simulink model "simulacion_controlador_lqr_entrada_velocidad"  (R2015a)
settings: Solver=ode45  StartTime=0.0  StopTime=144  RelTol=1e-3
values from neighbouring files (symbols this model uses):
  g = 9.81    [bola_viga_funciones.m]    (also in bola_viga_vel_funciones.m)
  Ib = 0.4*m*R^2    (= 4.624e-05)    [bola_viga_funciones.m]    (also in bola_viga_vel_funciones.m)
  L1 = place(AD',(CD*AD)',Pzo)'    [bola_viga_funciones.m]    (also in bola_viga_vel_funciones.m)
  m = 0.1    [bola_viga_funciones.m]    (also in bola_viga_vel_funciones.m)
  R = 0.034    [bola_viga_funciones.m]    (also in bola_viga_vel_funciones.m)
  T = 0.06    [bola_viga_funciones.m]    (also in bola_viga_vel_funciones.m)
undefined symbols (not defined in the file or in its folder): AD, BD, CD, K1
libraries: simulink x2
settings Model: Creator=HAROLD  LastModifiedBy=HAROLD

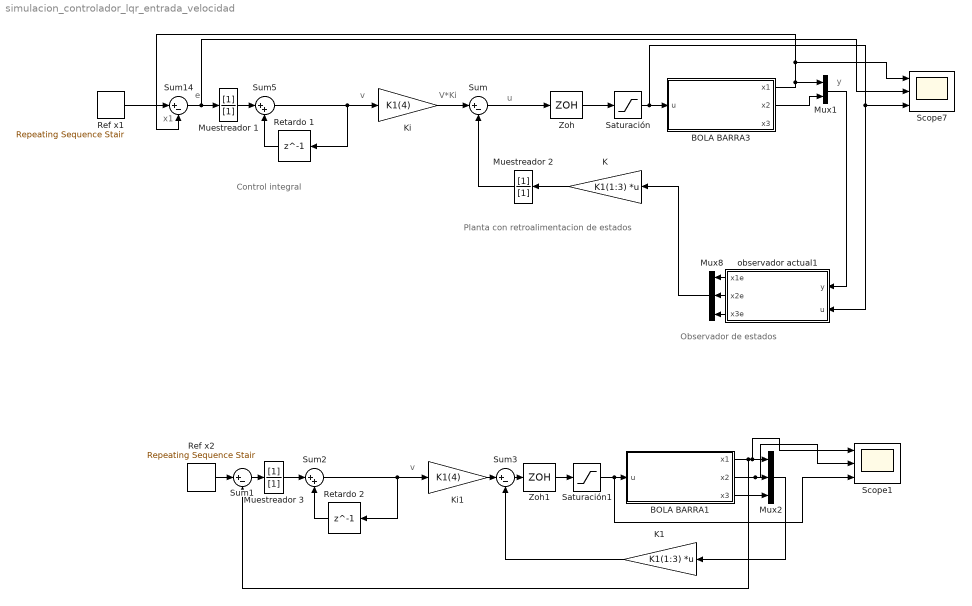
== system simulacion_controlador_lqr_entrada_velocidad ==
  note: x1
  note: V*Ki
  note: y
  note: u
  note: v
  note: e
  note: Planta con retroalimentacion de estados
  note: Control integral
  note: Observador de estados
  note: v
  BOLA BARRA1 : Subsystem
  BOLA BARRA3 : Subsystem
  K : Gain  Gain=K1(1:3)  Multiplication=Matrix(K*u)
  K1 : Gain  Gain=K1(1:3)  Multiplication=Matrix(K*u)
  Ki : Gain  Gain=K1(4)
  Ki1 : Gain  Gain=K1(4)
  Muestreador 1 : DiscreteFilter  Denominator=[1]  SampleTime=T
  Muestreador 2 : DiscreteFilter  Denominator=[1]  SampleTime=T
  Muestreador 3 : DiscreteFilter  Denominator=[1]  SampleTime=T
  Mux1 : Mux  Inputs=2
  Mux2 : Mux  Inputs=3
  Mux8 : Mux  Inputs=3
  Ref x1 : simulink/Sources/Repeating Sequence Stair  OutValues="[0.2  0.4 -0.4 -0.1 -0.3].'"  tsamp=36*0.8  OutMin=[]  OutMax=[]  OutDataTypeStr=double  OutputDataTypeScalingMode=double  OutDataType=fixdt(0,8)  ConRadixGroup=Best Precision: Vector-wise  OutScaling=2^-12
  Ref x2 : simulink/Sources/Repeating Sequence Stair  OutValues="[0.2  0.4 -0.4 -0.1 -0.3].'"  tsamp=36  OutMin=[]  OutMax=[]  OutDataTypeStr=double  OutputDataTypeScalingMode=double  OutDataType=fixdt(0,8)  ConRadixGroup=Best Precision: Vector-wise  OutScaling=2^-12
  Retardo 1 : Delay  DelayLength=1  SampleTime=T
  Retardo 2 : Delay  DelayLength=1  SampleTime=T
  Saturación : Saturate  UpperLimit=2.11  LowerLimit=-2.11
  Saturación1 : Saturate  UpperLimit=2.11  LowerLimit=-2.11
  Scope1 : Scope  NumInputPorts=3
      settings: YMin=-5~-5~-5  YMax=5~5~5  SaveName=datos
  Scope7 : Scope  NumInputPorts=3
      settings: YMin=-5~-5~-5  YMax=5~5~5  SaveName=datos1
  Sum{,1,3,14} (4 alike) : Sum  Inputs=|+-
  Sum2 : Sum  Inputs=|++
  Sum5 : Sum  Inputs=|++
  Zoh : ZeroOrderHold  SampleTime=T
  Zoh1 : ZeroOrderHold  SampleTime=T
  observador actual1 : Subsystem
  wires:
  K/1 -> Muestreador 2/1
  Zoh/1 -> Saturación/1
  Sum14/1 -> Scope7/2, Muestreador 1/1
  Retardo 1/1 -> Sum5/2
  Sum5/1 -> Retardo 1/1, Ki/1
  Ki/1 -> Sum/1
  Muestreador 1/1 -> Sum5/1
  Ref x1/1 -> Sum14/1
  Muestreador 2/1 -> Sum/2
  BOLA BARRA3/1(x1) -> Scope7/1, Sum14/2, Mux1/1
  Saturación/1 -> observador actual1/2(u), Scope7/3, BOLA BARRA3/1(u)
  observador actual1/1(x1e) -> Mux8/1
  observador actual1/2(x2e) -> Mux8/2
  Mux8/1 -> K/1
  BOLA BARRA3/2(x2) -> Mux1/2
  Mux1/1 -> observador actual1/1(y)
  Sum/1 -> Zoh/1
  observador actual1/3(x3e) -> Mux8/3
  Ref x2/1 -> Sum1/1
  Retardo 2/1 -> Sum2/2
  Sum2/1 -> Retardo 2/1, Ki1/1
  Muestreador 3/1 -> Sum2/1
  Sum1/1 -> Muestreador 3/1
  Ki1/1 -> Sum3/1
  K1/1 -> Sum3/2
  Zoh1/1 -> Saturación1/1
  Sum3/1 -> Zoh1/1
  Saturación1/1 -> Scope1/3, BOLA BARRA1/1(u)
  BOLA BARRA1/1(x1) -> Sum1/2, Scope1/1, Mux2/1
  BOLA BARRA1/2(x2) -> Scope1/2, Mux2/2
  BOLA BARRA1/3(x3) -> Mux2/3
  Mux2/1 -> K1/1

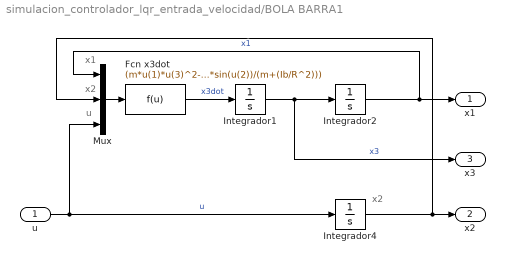
== system simulacion_controlador_lqr_entrada_velocidad/BOLA BARRA1 ==
  note: u
  note: x2
  note: x1
  note: x2
  u : Inport
  Fcn x3dot : Fcn  Expr=(m*u(1)*u(3)^2-m*g*sin(u(2))/(m+(Ib/R^2)))
  Integrador1 : Integrator
  Integrador2 : Integrator  InitialCondition=-10.2e-3
  Integrador4 : Integrator
  Mux : Mux  Inputs=3
  x1 : Outport
  x2 : Outport  Port=2
  x3 : Outport  Port=3
  wires:
  Integrador2/1 -> Mux/1, x1/1  "x1"
  Mux/1 -> Fcn x3dot/1
  Integrador1/1 -> x3/1, Integrador2/1  "x3"
  Integrador4/1 -> Mux/2, x2/1
  Fcn x3dot/1 -> Integrador1/1  "x3dot"
  u/1 -> Mux/3, Integrador4/1  "u"

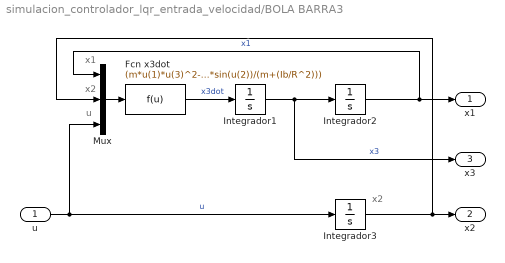
== system simulacion_controlador_lqr_entrada_velocidad/BOLA BARRA3 ==
  note: u
  note: x2
  note: x1
  note: x2
  u : Inport
  Fcn x3dot : Fcn  Expr=(m*u(1)*u(3)^2-m*g*sin(u(2))/(m+(Ib/R^2)))
  Integrador1 : Integrator
  Integrador2 : Integrator
  Integrador3 : Integrator
  Mux : Mux  Inputs=3
  x1 : Outport
  x2 : Outport  Port=2
  x3 : Outport  Port=3
  wires:
  Integrador2/1 -> Mux/1, x1/1  "x1"
  Mux/1 -> Fcn x3dot/1
  Integrador1/1 -> x3/1, Integrador2/1  "x3"
  Integrador3/1 -> Mux/2, x2/1
  Fcn x3dot/1 -> Integrador1/1  "x3dot"
  u/1 -> Mux/3, Integrador3/1  "u"

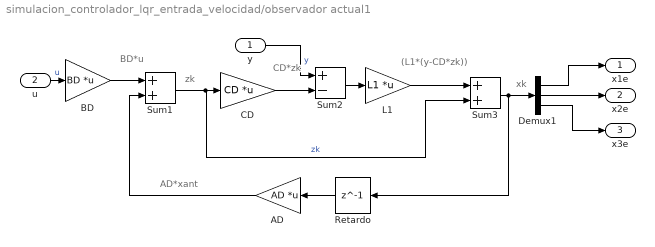
== system simulacion_controlador_lqr_entrada_velocidad/observador actual1 ==
  note: xk
  note: (L1*(y-CD*zk))
  note: CD*zk
  note: AD*xant
  note: BD*u
  note: zk
  y : Inport
  u : Inport  Port=2
  AD : Gain  Gain=AD  Multiplication=Matrix(K*u)
  BD : Gain  Gain=BD  Multiplication=Matrix(K*u)
  CD : Gain  Gain=CD  Multiplication=Matrix(K*u)
  Demux1 : Demux  Outputs=3
  L1 : Gain  Gain=L1  Multiplication=Matrix(K*u)
  Retardo : Delay  DelayLength=1  InitialCondition=[0 0 0]  SampleTime=T
  Sum1 : Sum
  Sum2 : Sum  Inputs=+-
  Sum3 : Sum
  x1e : Outport
  x2e : Outport  Port=2
  x3e : Outport  Port=3
  wires:
  Demux1/1 -> x1e/1
  Demux1/2 -> x2e/1
  Demux1/3 -> x3e/1
  Sum2/1 -> L1/1
  Sum1/1 -> Sum3/2, CD/1  "zk"
  Sum3/1 -> Demux1/1, Retardo/1
  BD/1 -> Sum1/1
  AD/1 -> Sum1/2
  L1/1 -> Sum3/1
  CD/1 -> Sum2/2
  Retardo/1 -> AD/1
  u/1 -> BD/1  "u"
  y/1 -> Sum2/1  "y"
